simulink model "SiEngineController"  (R2021a)
settings: Solver=ode4  StartTime=0.0  StopTime=inf  FixedStep=.01  RelTol=1e-3  EnableMultiTasking=on
model workspace (MAT data in the model file):
  CatLightOffTime = 0
  Cps = 2
  CrankSpeed = 150
  EngRevLim = 7000
  EngStopStartEnable = 1
  EngStopTime = Simulink.Parameter
  EngStopTime.Value = 5
  EngStopTime.DataType = 'auto'
  EngStopTime.Dimensions = [1 1]
  NCyl = 4
  N_idle = 750
  Pstd = 101325
  Rair = 287
  Sinj = 6.45161290323
  Ts = Simulink.Parameter
  Ts.Value = 0.01
  Ts.DataType = 'auto'
  Ts.Dimensions = [1 1]
  Tstd = 293.15
  Vd = 0.0015
  afr_stoich = 14.6
  calEngVar.core.f_lcmd = [0 0.191691264188 0.286571334902 0.358602176134 0.434951283804 0.517809198874 0.591334436539 0.614814588717 0.614814588717 0.614814588717 0.614814588717 0.614814588717 ... (315 elements, 21x15)]
  calEngVar.core.f_tap = [0 0.526932471044 0.76956291542 0.98216380025 1.2334307097 1.55068264267 2.00046965195 2.58135641722 2.62499999998 2.62499999998 2.62499999998 2.62499999998 ... (315 elements, 21x15)]
  calEngVar.core.f_wap = [100 100 100 100 100 100 100 100 100 100 100 100 ... (315 elements, 21x15)]
  calEngVar.coreNA.f_lcmd = [0 0.191673794394 0.286578553279 0.358630611212 0.435152304136 0.517511359701 0.591296787037 0.615501202156 0.615501210228 0.615501210228 0.615501210228 0.615501210228 ... (315 elements, 21x15)]
  calEngVar.coreNA.f_tap = [0 0.527345235487 0.765291494628 0.982320090429 1.22180310315 1.45741501873 1.75117231993 2.09744444378 2.125 2.125 2.125 2.125 ... (315 elements, 21x15)]
  calEngVar.coreNA.f_wap = [100 100 100 100 100 100 100 100 100 100 100 100 ... (315 elements, 21x15)]
  calEngVar.coreV.f_lcmd = [0 0.19142142175 0.28657735538 0.358588533041 0.434930199402 0.517764999878 0.59133168275 0.613384909963 0.613384909963 0.613384909963 0.613384909963 0.613384909963 ... (315 elements, 21x15)]
  calEngVar.coreV.f_tap = [0 0.527863235367 0.770830079631 0.984101120968 1.23616152686 1.5569502711 2.00981324054 2.59638620578 2.62499999998 2.62499999998 2.62499999998 2.62499999998 ... (315 elements, 21x15)]
  calEngVar.coreV.f_wap = [100 100 100 100 100 100 100 100 100 100 100 100 ... (315 elements, 21x15)]
  calEngVar.coreV2.f_lcmd = [0 0.194061751811 0.287076886903 0.3590121815 0.434856377449 0.517000734972 0.591338875255 0.631368486456 0.631368659193 0.631369289149 0.631369867036 0.631370221687 ... (315 elements, 21x15)]
  calEngVar.coreV2.f_tap = [0 0.39343253598 0.590588334546 0.770979852779 0.943173252011 1.20206320745 1.55415450545 2.04859058792 2.24999782819 2.24999782819 2.24999782819 2.24999782819 ... (315 elements, 21x15)]
  calEngVar.coreV2.f_wap = [100 100 100 100 100 100 100 100 100 100 100 100 ... (315 elements, 21x15)]
  calEngVar.coreVNA.f_lcmd = [0 0.191673794061 0.286578553391 0.358630612358 0.435152307947 0.517511360226 0.591296786776 0.615501114385 0.615501127394 0.615501127394 0.615501127394 0.615501127394 ... (315 elements, 21x15)]
  calEngVar.coreVNA.f_tap = [0 0.527345232618 0.765291631754 0.982320090196 1.22180322428 1.45741497917 1.75117250183 2.09744443735 2.125 2.125 2.125 2.125 ... (315 elements, 21x15)]
  calEngVar.coreVNA.f_wap = [100 100 100 100 100 100 100 100 100 100 100 100 ... (315 elements, 21x15)]
  f_cp_ld_bpt = [0 0.2 0.275 0.35 0.425 0.5 0.575 0.65 0.725 0.8 0.875 0.95 1.025 1.1 1.175 1.25]
  f_cp_n_bpt = [750 1053.57142857 1357.14285714 1660.71428571 1964.28571429 2267.85714286 2571.42857143 2875 3178.57142857 3482.14285714 3785.71428571 4089.28571429 4392.85714286 4696.42857143 5000]
  f_del_sa_bpt = [0 0.75 1.5 2.25 3 3.75 4.5 5.25 6 6.75 7.5 8.25 9 9.75 10.5 11.25 12 12.75 13.5 14.25 15 15.75 16.5 17.25 18 18.75 19.5 20.25 21 21.75 22.5 23.25 24 24.75 25.5 26.25 27 27.75 28.5 29.25 30 30.75 31.5 32.25 33 33.75 34.5 35.25 36 36.75 37.5 38.25 39 39.75 40.5 41.25 42 42.75 43.5 44.25 45 45.75 46.5 47.25 48]
  f_ecp = [0 0 7.19012817097 15.3709456879 19.1470470057 19.0854874367 13.5819971805 0 0 0 0 0 ... (240 elements, 16x15)]
  f_egr_areapct_cmd = [0 3.448 6.897 10.34 13.79 17.24 20.69 24.14 27.59 31.03 34.48 37.93 ... (600 elements, 30x20)]
  f_egr_areapct_nrmlzdflow_bpt = [0 0.03448 0.06897 0.1034 0.1379 0.1724 0.2069 0.2414 0.2759 0.3103 0.3448 0.3793 0.4138 0.4483 0.4828 0.5172 0.5517 0.5862 0.6207 0.6552 0.6897 0.7241 0.7586 0.7931 0.8276 0.8621 0.8966 0.931 0.9655 1]
  f_egr_areapct_pr_bpt = [0.5; 0.5263; 0.5526; 0.5789; 0.6053; 0.6316; 0.6579; 0.6842; 0.7105; 0.7368; 0.7632; 0.7895; 0.8158; 0.8421; 0.8684; 0.8947; 0.9211; 0.9474; 0.9737; 1]
  f_egr_max_stdflow = [74.87 74.87 74.74 74.39 73.81 72.98 71.91 70.58 68.97 67.06 64.84 62.25 59.27 55.81 51.79 47.07 36.33 24.22 12.11 0]
  f_egr_stdflow = [0 3.743 7.487 11.23 14.97 18.72 22.46 26.2 29.95 33.69 37.43 41.18 ... (420 elements, 21x20)]
  f_egr_stdflow_egrap_bpt = [0; 5; 10; 15; 20; 25; 30; 35; 40; 45; 50; 55; 60; 65; 70; 75; 80; 85; 90; 95; 100]
  f_egr_stdflow_pr_bpt = [0.5; 0.5263; 0.5526; 0.5789; 0.6053; 0.6316; 0.6579; 0.6842; 0.7105; 0.7368; 0.7632; 0.7895; 0.8158; 0.8421; 0.8684; 0.8947; 0.9211; 0.9474; 0.9737; 1]
  f_egrpct_cmd = [0  0  0  0  0  0  0  0  0  0  0  0  0  0  0; 0  0  0  0  0  0  0  0  0  0  0  0  0  0  0; 0  0  0  0  0  0  0  0  0  0  0  0  0  0  0; 0  0  0  0  0  0  0  0  0  0  0  0  0  0  0; 0  0  0  0  0  0  0  0  0  0  0  0  0  0  0; 0  0  0  0  0  0  0  0  0  0  0  0  0  0  0; 0  0  0  0  0  0  0  0  0  0  0  0  0  0  0; 0  0  0  0  0  0  0  0  0  0  0  0  0  0  0; 0  0  0  0  0  0  0  0  0  0  0  0  0  0  0; 0  0  0  0  0  0  0  0  0  0  0  0  0  0  0; 0  0  0  0  0  0  0  0  0  0  0  0  0  0  0; 0  0  0  0  0  0  0  0  0  0  0  0  0  0  0; 0  0  0  0  0  0  0  0  0  0  0  0  0  0  0; 0  0  0  0  0  0  0  0  0  0  0  0  0  0  0; 0  0  0  0  0  0  0  0  0  0  0  0  0  0  0; 0  0  0  0  0  0  0  0  0  0  0  0  0  0  0]
  f_egrpct_ld_bpt = [0 0.2 0.275 0.35 0.425 0.5 0.575 0.65 0.725 0.8 0.875 0.95 1.025 1.1 1.175 1.25]
  f_egrpct_n_bpt = [750 1054 1357 1661 1964 2268 2571 2875 3179 3482 3786 4089 4393 4696 5000]
  f_fric_temp_bpt = [274 276 278 280 282 284 286 288 290 292 294 296 298 300 302 304 306 308 310 312 314 316 318 320 322 324 326 328 330 332 334 336 338 340 342 344 346 348 350 352 354 356 358 360 362 364 366 368 370 372 374 376 378 380]
  f_fric_temp_mod = [3.96 3.22 2.56 2.26 2.11 2 1.9 1.83 1.76 1.7 1.65 1.6 1.55 1.49 1.44 1.41 1.38 1.35 1.32 1.3 1.27 1.25 1.24 1.21 1.2 1.18 1.16 1.15 1.13 1.12 1.11 1.1 1.09 1.08 1.07 1.06 1.05 1.05 1.04 1.03 1.02 1.02 1.01 1.01 1 1 1 0.999 0.997 0.995 0.993 0.991 0.989 0.987]
  f_icp = [0 0 1 1.09273642197 2.29409401139 3.54274371837 0.947749647567 0 0 0 0 0 ... (240 elements, 16x15)]
  f_intksys_stdflow_bpt = [0 29.67 59.34 89.01 117.8 144.1 155.7 166 175.2 183.3 190.7 197 202.7 207.7 212.2 216.1 219.4 222.2 224.5 226.4]
  f_intksys_stdflow_pr = [1 0.9789 0.9579 0.9368 0.9158 0.8947 0.8737 0.8526 0.8316 0.8105 0.7895 0.7684 0.7474 0.7263 0.7053 0.6842 0.6632 0.6421 0.6211 0.6]
  f_lamcmd = [1  1  1  1  1  1  1  1  1  1  1  1  1  1  1; 1  1  1  1  1  1  1  1  1  1  1  1  1  1  1; 1  1  1  1  1  1  1  1  1  1  1  1  1  1  1; 1  1  1  1  1  1  1  1  1  1  1  1  1  1  1; 1  1  1  1  1  1  1  1  1  1  1  1  1  1  1; 1  1  1  1  1  1  1  1  1  1  1  1  1  1  1; 1  1  1  1  1  1  1  1  1  1  1  1  1  1  1; 1  1  1  1  1  1  1  1  1  1  1  1  1  1  1; 1  1  1  1  1  1  1  1  1  1  1  1  1  1  1; 1  1  1  1  1  1  1  1  1  1  1  1  1  1  1; 1  1  1  1  1  1  1  1  1  1  1  1  1  1  0.978833376279; 1  1  1  1  1  0.994115442909  1  0.972947102204  0.980523305065  0.999379925377  1  0.999606769395  0.999730304812  0.995941175028  0.966904774685; 1  1  1  0.94651624294  1  0.952506105741  0.994491417815  0.906466250495  0.924122061249  0.974767007025  0.985748891861  0.982416523617  0.992900047913  0.942109771144  0.941787575943; 1  1  1  0.942  0.937279637266  0.910896768573  0.929830385386  0.839985398785  0.854904769548  0.889462296842  0.92380217143  0.919912974116  0.958707785886  0.945711085936  0.914402970615; 1  1  1  0.942  0.902  0.869287431405  0.865169352957  0.81  0.824  0.812  0.837314196571  0.85940898562  0.888506841156  0.882667105929  0.87548189152; 1  1  1  0.942  0.902  0.846  0.824  0.81  0.824  0.812  0.826  0.818  0.815209011399  0.813810193086  0.836]
  f_lamcmd_ld_bpt = [0 0.2 0.275 0.35 0.425 0.5 0.575 0.65 0.725 0.8 0.875 0.95 1.025 1.1 1.175 1.25]
  f_lamcmd_n_bpt = [750 1053.57142857 1357.14285714 1660.71428571 1964.28571429 2267.85714286 2571.42857143 2875 3178.57142857 3482.14285714 3785.71428571 4089.28571429 4392.85714286 4696.42857143 5000]
  f_lcmd = [0 0.191691264188 0.286571334902 0.358602176134 0.434951283804 0.517809198874 0.591334436539 0.614814588717 0.614814588717 0.614814588717 0.614814588717 0.614814588717 ... (315 elements, 21x15)]
  f_lcmd_n_bpt = [750 1053.57142857 1357.14285714 1660.71428571 1964.28571429 2267.85714286 2571.42857143 2875 3178.57142857 3482.14285714 3785.71428571 4089.28571429 4392.85714286 4696.42857143 5000]
  f_lcmd_tq_bpt = [0 15 26.3157894737 37.6315789474 48.9473684211 60.2631578947 71.5789473684 82.8947368421 94.2105263158 105.526315789 116.842105263 128.157894737 139.473684211 150.789473684 162.105263158 173.421052632 184.736842105 196.052631579 207.368421053 218.684210526 230]
  f_m_lam = [0.94128 0.95565 0.97001 0.98437 0.99008 1.0004 0.97527 0.9549 0.92612 0.89735 0]
  f_m_lam_bpt = [0.65 0.7 0.75 0.8 0.85 0.9 0.95 1 1.05 1.1 2]
  f_m_sa = [1.0019 0.9988 0.9953 0.99173 0.98811 0.98441 0.98065 0.97682 0.97293 0.96897 0.96493 0.96083 0.95666 0.95242 0.94811 0.94373 0.93927 0.93475 0.93015 0.92548 0.92074 0.91592 0.91104 0.90608 0.90105 0.89594 0.89076 0.88551 0.88019 0.8748 0.86933 0.86379 0.85818 0.8525 0.84675 0.84093 0.83503 0.82907 0.82303 0.81693 0.81075 0.80451 0.79819 0.79181 0.78536 0.77884 0.77226 0.7656 0.75888 0.75209 0.74524 0.73832 0.73134 0.72429 0.71717 0.70999 0.70275 0.69682 0.68949 0.68303 0.67548 0.67037 0.66525 0.66014 0.65503]
  f_mdot_air_corr = [1.02156051768 1.00597426471 0.989411677851 1.0033499089 0.984591437857 0.988509040623 1.0326198627 1.02765527362 1.0134784519 0.998280021213 0.981755128787 0.967218261288 ... (400 elements, 20x20)]
  f_mdot_air_corr_ld_bpt = [0.223381333333 0.285105122807 0.346828912281 0.408552701754 0.470276491228 0.532000280702 0.593724070175 0.655447859649 0.717171649123 0.778895438596 0.84061922807 0.902343017544 0.964066807018 1.02579059649 1.08751438596 1.14923817544 1.21096196491 1.27268575439 1.33440954386 1.39613333333]
  f_mdot_air_n_bpt = [750 973.6842 1197.3684 1421.0526 1644.7368 1868.4211 2092.1053 2315.7895 2539.4737 2763.1579 2986.8421 3210.5263 3434.2105 3657.8947 3881.5789 4105.2632 4328.9474 4552.6316 4776.3158 5000]
  f_mdot_intk = [0 0 0 0 0 0 0 0 0 0 0 0 ... (400 elements, 20x20)]
  f_mdot_intk_ecp_bpt = [0 2.6316 5.2632 7.8947 10.5263 13.1579 15.7895 18.4211 21.0526 23.6842 26.3158 28.9474 31.5789 34.2105 36.8421 39.4737 42.1053 44.7368 47.3684 50]
  f_mdot_trpd_bpt = [0 5.7895 11.5789 17.3684 23.1579 28.9474 34.7368 40.5263 46.3158 52.1053 57.8947 63.6842 69.4737 75.2632 81.0526 86.8421 92.6316 98.4211 104.2105 110]
  f_nv = [0.64175366561 0.641419295169 0.640125365558 0.638690556197 0.644169906538 0.669178791311 0.731659452876 0.750078238889 0.750078238889 0.750078238889 0.750078238889 0.750078238889 ... (225 elements, 15x15)]
  f_nv_n_bpt = [750 1053.57142857 1357.14285714 1660.71428571 1964.28571429 2267.85714286 2571.42857143 2875 3178.57142857 3482.14285714 3785.71428571 4089.28571429 4392.85714286 4696.42857143 5000]
  f_nv_prs_bpt = [31 40.6428571429 50.2857142857 59.9285714286 69.5714285714 79.2142857143 88.8571428571 98.5 108.142857143 117.785714286 127.428571429 137.071428571 146.714285714 156.357142857 166]
  f_sa = [9.05 9.05 16.4373253582 15.3405265461 13.6074880273 9.83352189562 3.89388784387 0 0 0 0 0 ... (240 elements, 16x15)]
  f_sa_ld_bpt = [0 0.2 0.275 0.35 0.425 0.5 0.575 0.65 0.725 0.8 0.875 0.95 1.025 1.1 1.175 1.25]
  f_sa_n_bpt = [750 1053.57142857 1357.14285714 1660.71428571 1964.28571429 2267.85714286 2571.42857143 2875 3178.57142857 3482.14285714 3785.71428571 4089.28571429 4392.85714286 4696.42857143 5000]
  f_sa_opt = [9.05 9.05 16.4373253582 15.3405265461 13.6074880273 9.83352189562 3.89388784387 2.22044604925e-16 2.22044604925e-16 2.22044604925e-16 2.22044604925e-16 2.22044604925e-16 ... (256 elements, 16x16)]
  f_startup_ect_bpt = [-40 0 20 50]
  f_startup_lambda_delta = [0.5 0.3 0.2 0]
  f_startup_lambda_delta_timecnst = [90 40 12 0]
  f_t_exh = [739.936218766 750.584766028 772.770773797 791.235245621 803.106549716 885.862998064 920.498479307 920.498479307 920.498479307 920.498479307 920.498479307 920.498479307 ... (225 elements, 15x15)]
  f_t_exh_l_bpt = [0.2 0.275 0.35 0.425 0.5 0.575 0.65 0.725 0.8 0.875 0.95 1.025 1.1 1.175 1.25]
  f_t_exh_n_bpt = [750 1053.57142857 1357.14285714 1660.71428571 1964.28571429 2267.85714286 2571.42857143 2875 3178.57142857 3482.14285714 3785.71428571 4089.28571429 4392.85714286 4696.42857143 5000]
  f_tap = [0 0.526932471044 0.76956291542 0.98216380025 1.2334307097 1.55068264267 2.00046965195 2.58135641722 2.62499999998 2.62499999998 2.62499999998 2.62499999998 ... (315 elements, 21x15)]
  f_tap_ld_bpt = [0 0.2 0.268421052632 0.336842105263 0.405263157895 0.473684210526 0.542105263158 0.610526315789 0.678947368421 0.747368421053 0.815789473684 0.884210526316 0.952631578947 1.02105263158 1.08947368421 1.15789473684 1.22631578947 1.29473684211 1.36315789474 1.43157894737 1.5]
  f_tap_n_bpt = [750 1053.57142857 1357.14285714 1660.71428571 1964.28571429 2267.85714286 2571.42857143 2875 3178.57142857 3482.14285714 3785.71428571 4089.28571429 4392.85714286 4696.42857143 5000]
  f_tm_corr = [0.839360054391 0.833393271885 0.82629554201 0.818442814437 0.811524387436 0.809164184856 0.814606352881 0.826887956871 0.842304598924 0.856886829014 0.869487025783 0.880530414174 ... (400 elements, 20x20)]
  f_tm_corr_n_bpt = [750 973.6842 1197.3684 1421.0526 1644.7368 1868.4211 2092.1053 2315.7895 2539.4737 2763.1579 2986.8421 3210.5263 3434.2105 3657.8947 3881.5789 4105.2632 4328.9474 4552.6316 4776.3158 5000]
  f_tm_corr_nd_bpt = [0.3 0.38947 0.47895 0.56842 0.65789 0.74737 0.83684 0.92632 1.0158 1.1053 1.1947 1.2842 1.3737 1.4632 1.5526 1.6421 1.7316 1.8211 1.9105 2]
  f_tpp = [0 100]
  f_tpp_tap_bpt = [0 100]
  f_tq_fric = [0  4.16  4.8  5.44  6.05  6.64  7.23  7.81  8.39  8.97  9.54  10.1  10.7  11.3  11.9  12.5; 0  4.16  4.8  5.44  6.05  6.64  7.23  7.81  8.39  8.97  9.54  10.1  10.7  11.3  11.9  12.5; 0  4.42  5.07  5.69  6.29  6.89  7.49  8.09  8.69  9.28  9.86  10.4  11  11.6  12.2  12.8; 0  4.69  5.36  5.98  6.58  7.18  7.79  8.41  9.02  9.62  10.2  10.8  11.4  11.9  12.5  13.1; 0  4.88  5.59  6.25  6.87  7.48  8.09  8.71  9.32  9.92  10.5  11.1  11.7  12.3  12.9  13.4; 0  4.94  5.74  6.45  7.12  7.75  8.37  8.99  9.59  10.2  10.8  11.4  11.9  12.6  13.2  13.8; 0  4.93  5.76  6.56  7.29  7.97  8.62  9.23  9.83  10.4  11  11.6  12.2  12.8  13.4  14.1; 0  4.85  5.67  6.57  7.37  8.11  8.8  9.43  10  10.6  11.2  11.8  12.4  13  13.7  14.3; 0  4.74  5.57  6.46  7.34  8.14  8.88  9.55  10.2  10.8  11.4  12  12.6  13.2  13.8  14.4; 0  4.63  5.42  6.27  7.19  8.05  8.83  9.55  10.2  10.9  11.5  12.1  12.7  13.3  14  14.6; 0  4.52  5.29  6.11  6.98  7.84  8.65  9.4  10.1  10.8  11.5  12.1  12.8  13.4  14.1  14.6; 0  4.42  5.18  5.97  6.79  7.6  8.39  9.15  9.88  10.6  11.3  12.1  12.8  13.5  14.1  14.7; 0  4.34  5.09  5.86  6.64  7.42  8.17  8.88  9.6  10.3  11.1  11.9  12.7  13.4  14.1  14.7; 0  4.27  5.01  5.76  6.52  7.28  8.03  8.74  9.39  10.1  10.8  11.6  12.4  13.2  14  14.7; 0  4.21  4.94  5.67  6.42  7.16  7.89  8.59  9.25  9.93  10.7  11.5  12.3  13.1  13.8  14.6; 0  4.15  4.87  5.6  6.33  7.06  7.77  8.47  9.14  9.84  10.6  11.3  12.1  12.9  13.7  14.4]
  f_tq_inr = [25.8508 25.8508 31 37 43 50 50 50 50 50 50 50 ... (256 elements, 16x16)]
  f_tq_inr_l_bpt = [0.1 0.2 0.28571 0.37143 0.45714 0.54286 0.62857 0.71429 0.8 0.88571 0.97143 1.0571 1.1429 1.2286 1.3143 1.4]
  f_tq_inr_n_bpt = [0 750 1053.5714 1357.1429 1660.7143 1964.2857 2267.8571 2571.4286 2875 3178.5714 3482.1429 3785.7143 4089.2857 4392.8571 4696.4286 5000]
  f_tq_nl = [0 15.0012133443 26.4298333923 37.8556656512 49.2846782956 60.7113978793 72.3451969202 77.459652163 78.5324534074 78.5324534074 78.5324534074 78.5324534074 ... (256 elements, 16x16)]
  f_tq_nl_l_bpt = [0 0.2 0.275 0.35 0.425 0.5 0.575 0.65 0.725 0.8 0.875 0.95 1.025 1.1 1.175 1.25]
  f_tq_nl_n_bpt = [0 750 1053.57142857 1357.14285714 1660.71428571 1964.28571429 2267.85714286 2571.42857143 2875 3178.57142857 3482.14285714 3785.71428571 4089.28571429 4392.85714286 4696.42857143 5000]
  f_tq_pump = [0  7.24  7.7  7.82  7.95  8.1  8.27  8.45  8.64  8.78  8.88  8.96  9.03  9.12  9.25  9.45; 0  7.24  7.7  7.82  7.95  8.1  8.27  8.45  8.64  8.78  8.88  8.96  9.03  9.12  9.25  9.45; 0  5.67  6.03  6.37  6.67  6.92  7.14  7.33  7.5  7.67  7.84  8.01  8.19  8.38  8.58  8.8; 0  3.94  4.52  5  5.36  5.6  5.77  5.92  6.1  6.35  6.67  7.02  7.4  7.75  8.06  8.34; 0  2.59  3.14  3.57  3.86  4.05  4.21  4.43  4.76  5.21  5.75  6.32  6.85  7.3  7.65  7.92; 0  1.8  2.25  2.61  2.88  3.11  3.37  3.71  4.17  4.74  5.36  5.96  6.49  6.91  7.23  7.46; 0  1  1.36  1.77  2.15  2.51  2.88  3.31  3.8  4.37  4.98  5.57  6.11  6.57  6.94  7.25; 0  1  1  1  1.09  1.59  2.08  2.6  3.17  3.81  4.49  5.19  5.85  6.44  6.92  7.29; 0  1  1  1  1  1  1.62  2.32  3.05  3.83  4.64  5.44  6.19  6.82  7.31  7.65; 0  1  1  1  1  1  1.35  2.21  3.08  3.97  4.88  5.78  6.64  7.41  8.06  8.58; 0  1  1  1  1  1  1  1.77  2.67  3.58  4.55  5.6  6.73  7.91  9.07  10.1; 0  1  1  1  1  1  1  1.72  2.67  3.61  4.62  5.79  7.15  8.69  10.3  11.9; 0  1  1  1  1  1  1  1.74  2.88  3.96  5.08  6.36  7.86  9.57  11.4  13.2; 0  1  1  1  1  1  1  1.37  2.7  4.01  5.39  6.92  8.65  10.5  12.4  14.2; 0  1  1  1  1  1  1  1.28  2.66  4.14  5.72  7.43  9.28  11.2  13.1  14.8; 0  1  1  1  1  1  1  1.39  2.82  4.39  6.06  7.85  9.73  11.6  13.5  15.1]
  f_vivc = [0.37716 0.38164 0.38611 0.39033 0.39428 0.39795 0.40132 0.40441 0.40719 0.40967 0.41184 0.41372 0.41529 0.41656 0.41755 0.41825 0.41867 0.41884 0.41874 0.41865]
  f_vivc_icp_bpt = [0 2.6316 5.2632 7.8947 10.5263 13.1579 15.7895 18.4211 21.0526 23.6842 26.3158 28.9474 31.5789 34.2105 36.8421 39.4737 42.1053 44.7368 47.3684 50]
  f_wap = [100 100 100 100 100 100 100 100 100 100 100 100 ... (315 elements, 21x15)]
  f_wap_ld_bpt = [0 0.2 0.268421052632 0.336842105263 0.405263157895 0.473684210526 0.542105263158 0.610526315789 0.678947368421 0.747368421053 0.815789473684 0.884210526316 0.952631578947 1.02105263158 1.08947368421 1.15789473684 1.22631578947 1.29473684211 1.36315789474 1.43157894737 1.5]
  f_wap_n_bpt = [750 1053.57142857 1357.14285714 1660.71428571 1964.28571429 2267.85714286 2571.42857143 2875 3178.57142857 3482.14285714 3785.71428571 4089.28571429 4392.85714286 4696.42857143 5000]
  tau_egr = 0.2
libraries: simulink x3, autolibengctrlr x1
(part 1 of 2)
settings Model: ModifiedByFormat=The MathWorks, Inc.  OrderedModelArguments=off  Creator=The MathWorks, Inc.  LastModifiedBy=The MathWorks, Inc.
settings SolverCC: AlgebraicLoopSolver=TrustRegion
settings DataIOCC: DSMLogging=off  ReturnWorkspaceOutputs=off
settings DebuggingCC: PregeneratedLibrarySubsystemCodeDiagnostic=none  SFMachineParentedDataDiag=warning  ArithmeticOperatorsInVariantConditions=warning
settings SFSimCC: SimUseLocalCustomCode=off
settings RTWCC: RTWUseLocalCustomCode=off
settings CodeAppCC: StateflowObjectComments=on
settings GRTTargetCC: TargetLangStandard=C89/C90 (ANSI)
settings ConfigComp: CovMetricSettings=dsw  CovSaveCumulativeToWorkspaceVar=on  CovSaveSingleToWorkspaceVar=on  CovExternalEMLEnable=off

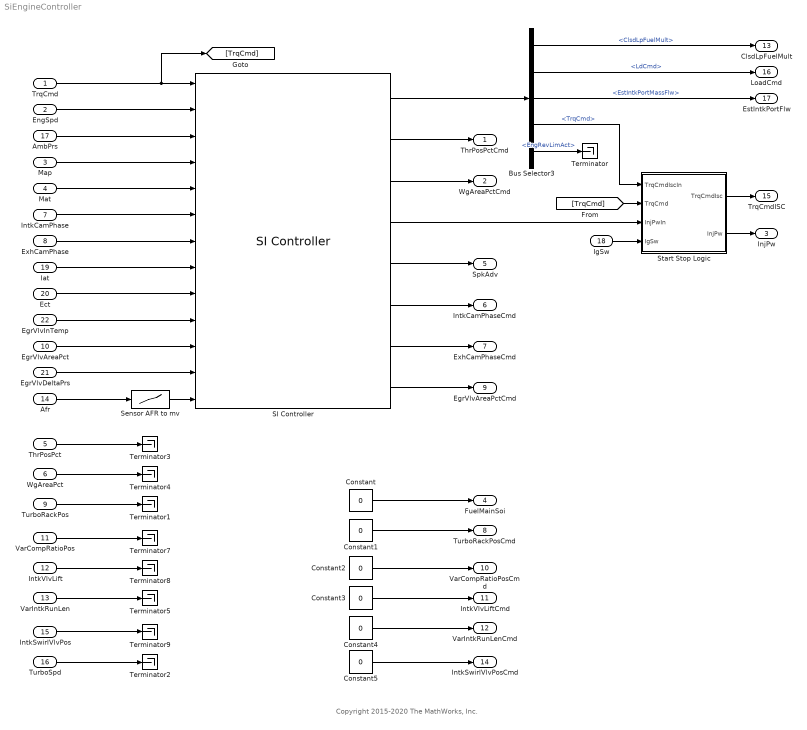
== system SiEngineController ==
  note: Copyright 2015-2020 The MathWorks, Inc.
  TrqCmd : Inport
  EngSpd : Inport  Port=2
  Map : Inport  Port=3
  Mat : Inport  Port=4
  ThrPosPct : Inport  Port=5  Unit=%
  WgAreaPct : Inport  Port=6  Unit=%
  IntkCamPhase : Inport  Port=7
  ExhCamPhase : Inport  Port=8
  TurboRackPos : Inport  Port=9  Unit=1
  EgrVlvAreaPct : Inport  Port=10  Unit=%
  VarCompRatioPos : Inport  Port=11
  IntkVlvLift : Inport  Port=12
  VarIntkRunLen : Inport  Port=13
  Afr : Inport  Port=14  Unit=1
  IntkSwirlVlvPos : Inport  Port=15
  TurboSpd : Inport  Port=16  Unit=rpm
  AmbPrs : Inport  Port=17
  IgSw : Inport  Port=18
  Iat : Inport  Port=19  Unit=K
  Ect : Inport  Port=20  Unit=K
  EgrVlvDeltaPrs : Inport  Port=21  Unit=Pa
  EgrVlvInTemp : Inport  Port=22  Unit=K
  Bus Selector3 : BusSelector  OutputSignals=ClsdLpFuelMult,LdCmd,EstIntkPortMassFlw,TrqCmd,EngRevLimAct
  Constant{,1..5} (6 alike) : Constant  Value=0  SampleTime=-1
  SI Controller : autolibengctrlr/SI Controller  AirEstOptionPopup=Dual Variable Cam Phasing  TrqEstOptionPopup=Torque Structure  f_lcmd=f_lcmd  f_lcmd_tq_bpt=f_lcmd_tq_bpt  f_lcmd_n_bpt=f_lcmd_n_bpt  f_tap=f_tap  f_tap_ld_bpt=f_tap_ld_bpt  f_tap_n_bpt=f_tap_n_bpt  f_tpp=f_tpp  f_tpp_tap_bpt=f_tpp_tap_bpt  f_wap=f_wap  f_wap_ld_bpt=f_wap_ld_bpt  f_wap_n_bpt=f_wap_n_bpt  f_icp=f_icp  f_ecp=f_ecp  f_cp_ld_bpt=f_cp_ld_bpt  f_cp_n_bpt=f_cp_n_bpt  f_egrpct_cmd=f_egrpct_cmd  f_egrpct_ld_bpt=f_egrpct_ld_bpt  f_egrpct_n_bpt=f_egrpct_n_bpt  f_egr_areapct_cmd=f_egr_areapct_cmd  f_egr_max_stdflow=f_egr_max_stdflow  f_egr_areapct_nrmlzdflow_bpt=f_egr_areapct_nrmlzdflow_bpt  f_egr_areapct_pr_bpt=f_egr_areapct_pr_bpt  LambdaCmdOvrd=off  Sinj=Sinj  Nmin=1  afr_stoich=afr_stoich  f_lamcmd=f_lamcmd  f_lamcmd_ld_bpt=f_lamcmd_ld_bpt  f_lamcmd_n_bpt=f_lamcmd_n_bpt  f_startup_lambda_delta=f_startup_lambda_delta  f_startup_lambda_delta_timecnst=f_startup_lambda_delta_timecnst  f_startup_ect_bpt=f_startup_ect_bpt  ClsdLpFuelEn=off  OpenLpDitherEn=off  LambdaDitherAmp=0.03  LambdaDitherFrq=0.75  ClsdLpFuelPGain=0.005  ClsdLpFuelIGain=0.05  ClsdLpFuelIntgLmt=0.2  O2ResetStoichVoltSen=2500  O2ResetMinVoltSen=0  O2ResetMaxVoltSen=5000  O2LearnUpdatePerSen=4  O2AmpMinVoltSen=250  O2ReadyVoltSen=1150  O2NotReadyVoltSen=1950  f_sa=f_sa  f_sa_ld_bpt=f_sa_ld_bpt  f_sa_n_bpt=f_sa_n_bpt  N_idle=N_idle  Trq_idlecmd_enable=1  Trq_idlecmd_max=50  Kp_idle=0.02  Ki_idle=0.01  EngRevLim=EngRevLim  CrankSpeed=CrankSpeed  NCyl=NCyl  Cps=Cps  Vd=Vd  Rair=Rair  Pstd=Pstd  Tstd=Tstd  f_nv=f_nv  f_nv_prs_bpt=f_nv_prs_bpt  f_nv_n_bpt=f_nv_n_bpt  f_vivc=f_vivc  f_tm_corr_n_bpt=f_tm_corr_n_bpt  f_vivc_icp_bpt=f_vivc_icp_bpt  f_tm_corr=f_tm_corr  f_tm_corr_nd_bpt=f_tm_corr_nd_bpt  f_mdot_intk=f_mdot_intk  f_mdot_intk_ecp_bpt=f_mdot_intk_ecp_bpt  f_mdot_trpd_bpt=f_mdot_trpd_bpt  f_mdot_air_corr=f_mdot_air_corr  f_mdot_air_corr_ld_bpt=f_mdot_air_corr_ld_bpt  f_mdot_air_n_bpt=f_mdot_air_n_bpt  tau_egr=tau_egr  f_intksys_stdflow_pr=f_intksys_stdflow_pr  f_intksys_stdflow_bpt=f_intksys_stdflow_bpt  f_egr_stdflow=f_egr_stdflow  f_egr_stdflow_pr_bpt=f_egr_stdflow_pr_bpt  f_egr_stdflow_egrap_bpt=f_egr_stdflow_egrap_bpt  f_tq_nl=f_tq_nl  f_tq_nl_l_bpt=f_tq_nl_l_bpt  f_tq_nl_n_bpt=f_tq_nl_n_bpt  f_tq_inr=f_tq_inr  f_tq_fric=f_tq_fric  f_fric_temp_mod=f_fric_temp_mod  f_fric_temp_bpt=f_fric_temp_bpt  f_tq_pump=f_tq_pump  f_sa_opt=f_sa_opt  f_tq_inr_l_bpt=f_tq_inr_l_bpt  f_tq_inr_n_bpt=f_tq_inr_n_bpt  f_m_sa=f_m_sa  f_del_sa_bpt=f_del_sa_bpt  f_m_lam=f_m_lam  f_m_lam_bpt=f_m_lam_bpt  f_t_exh=f_t_exh  f_t_exh_l_bpt=f_t_exh_l_bpt  f_t_exh_n_bpt=f_t_exh_n_bpt
      settings: SourceProductBaseCode=PW
  Sensor AFR to mv : Lookup  InputValues="[14.4540   14.6000   14.7460]"  Table="[950   450    50]"  LookUpMeth=Interpolation-Use End Values
  Start Stop Logic : Subsystem  TreatAsAtomicUnit=on
  Terminator{,1..5,7..9} (9 alike) : Terminator
  ThrPosPctCmd : Outport  VectorParamsAs1DForOutWhenUnconnected=off
  WgAreaPctCmd : Outport  Port=2  VectorParamsAs1DForOutWhenUnconnected=off
  InjPw : Outport  Port=3  Unit=ms  VectorParamsAs1DForOutWhenUnconnected=off
  FuelMainSoi : Outport  Port=4  Unit=deg  VectorParamsAs1DForOutWhenUnconnected=off
  SpkAdv : Outport  Port=5  VectorParamsAs1DForOutWhenUnconnected=off
  IntkCamPhaseCmd : Outport  Port=6  VectorParamsAs1DForOutWhenUnconnected=off
  ExhCamPhaseCmd : Outport  Port=7  VectorParamsAs1DForOutWhenUnconnected=off
  TurboRackPosCmd : Outport  Port=8  Unit=1  VectorParamsAs1DForOutWhenUnconnected=off
  EgrVlvAreaPctCmd : Outport  Port=9  Unit=%  VectorParamsAs1DForOutWhenUnconnected=off
  VarCompRatioPosCmd : Outport  Port=10  VectorParamsAs1DForOutWhenUnconnected=off
  IntkVlvLiftCmd : Outport  Port=11  VectorParamsAs1DForOutWhenUnconnected=off
  VarIntkRunLenCmd : Outport  Port=12  VectorParamsAs1DForOutWhenUnconnected=off
  ClsdLpFuelMult : Outport  Port=13  Unit=1  VectorParamsAs1DForOutWhenUnconnected=off
  IntkSwirlVlvPosCmd : Outport  Port=14  VectorParamsAs1DForOutWhenUnconnected=off
  TrqCmdISC : Outport  Port=15  Unit=N*m  VectorParamsAs1DForOutWhenUnconnected=off
  LoadCmd : Outport  Port=16  VectorParamsAs1DForOutWhenUnconnected=off
  EstIntkPortFlw : Outport  Port=17  VectorParamsAs1DForOutWhenUnconnected=off
  wires:
  AmbPrs/1 -> SI Controller/3
  Map/1 -> SI Controller/4
  Mat/1 -> SI Controller/5
  IntkCamPhase/1 -> SI Controller/6
  ExhCamPhase/1 -> SI Controller/7
  SI Controller/1 -> Bus Selector3/1
  SI Controller/4 -> Start Stop Logic/3(InjPwIn)
  Bus Selector3/4 -> Start Stop Logic/1(TrqCmdIscIn)  "<TrqCmd>"
  Constant1/1 -> TurboRackPosCmd/1
  EngSpd/1 -> SI Controller/2
  TrqCmd/1 -> SI Controller/1, [TrqCmd]
  Bus Selector3/3 -> EstIntkPortFlw/1  "<EstIntkPortMassFlw>"
  Bus Selector3/2 -> LoadCmd/1  "<LdCmd>"
  Constant/1 -> FuelMainSoi/1
  TurboRackPos/1 -> Terminator1/1
  TurboSpd/1 -> Terminator2/1
  Start Stop Logic/2(InjPw) -> InjPw/1
  [TrqCmd] -> Start Stop Logic/2(TrqCmd)
  Start Stop Logic/1(TrqCmdIsc) -> TrqCmdISC/1
  IntkSwirlVlvPos/1 -> Terminator9/1
  VarIntkRunLen/1 -> Terminator5/1
  IntkVlvLift/1 -> Terminator8/1
  VarCompRatioPos/1 -> Terminator7/1
  Constant5/1 -> IntkSwirlVlvPosCmd/1
  Constant4/1 -> VarIntkRunLenCmd/1
  Constant3/1 -> IntkVlvLiftCmd/1
  Constant2/1 -> VarCompRatioPosCmd/1
  ThrPosPct/1 -> Terminator3/1
  WgAreaPct/1 -> Terminator4/1
  SI Controller/6 -> IntkCamPhaseCmd/1
  SI Controller/7 -> ExhCamPhaseCmd/1
  SI Controller/5 -> SpkAdv/1
  SI Controller/2 -> ThrPosPctCmd/1
  SI Controller/3 -> WgAreaPctCmd/1
  IgSw/1 -> Start Stop Logic/4(IgSw)
  SI Controller/8 -> EgrVlvAreaPctCmd/1
  EgrVlvAreaPct/1 -> SI Controller/11
  EgrVlvDeltaPrs/1 -> SI Controller/12
  Iat/1 -> SI Controller/8
  EgrVlvInTemp/1 -> SI Controller/10
  Ect/1 -> SI Controller/9
  Bus Selector3/5 -> Terminator/1  "<EngRevLimAct>"
  Sensor AFR to mv/1 -> SI Controller/13
  Afr/1 -> Sensor AFR to mv/1
  Bus Selector3/1 -> ClsdLpFuelMult/1  "<ClsdLpFuelMult>"
